simulink model "Simulink_Model"  (R2023b)
settings: Solver=FixedStepAuto  StartTime=0.0  StopTime=100  FixedStep=1e-2  RelTol=1e-3
values from neighbouring files (symbols this model uses):
  A = pi*(diameter/2)^2    (= 0.0706858347058)    [param.m]
  C_d = 0.75    [param.m]
  dm_dt = 3    [param.m]
  h_0 = 0    [param.m]
  m_0 = 200    [param.m]
  m_fuel = 120    [param.m]
  v_exh = 900    [param.m]
undefined symbols (not defined in the file or in its folder): magnitude
libraries: cstblocks x1, simulink x1
settings Model: Creator=Aras Güngöre
settings SolverCC: AlgebraicLoopSolver=TrustRegion
settings DebuggingCC: UnconnectedInputMsg=warning  UnconnectedOutputMsg=warning  UnconnectedLineMsg=warning
settings ModelReferenceCC: EnableRefExpFcnMdlSchedulingChecks=on
settings RTWCC: DLArmComputeVersion=19.05

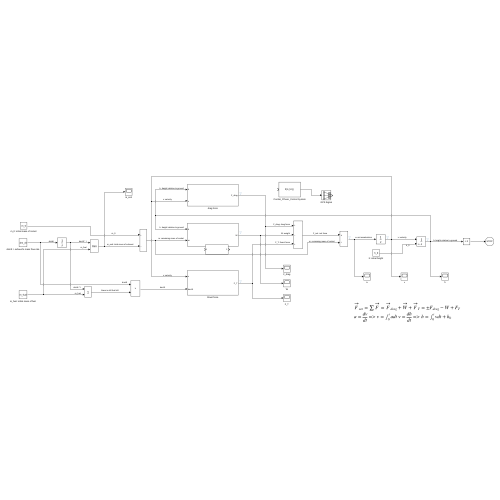
[thumbnail: Simulink's stored preview of the top-level diagram]
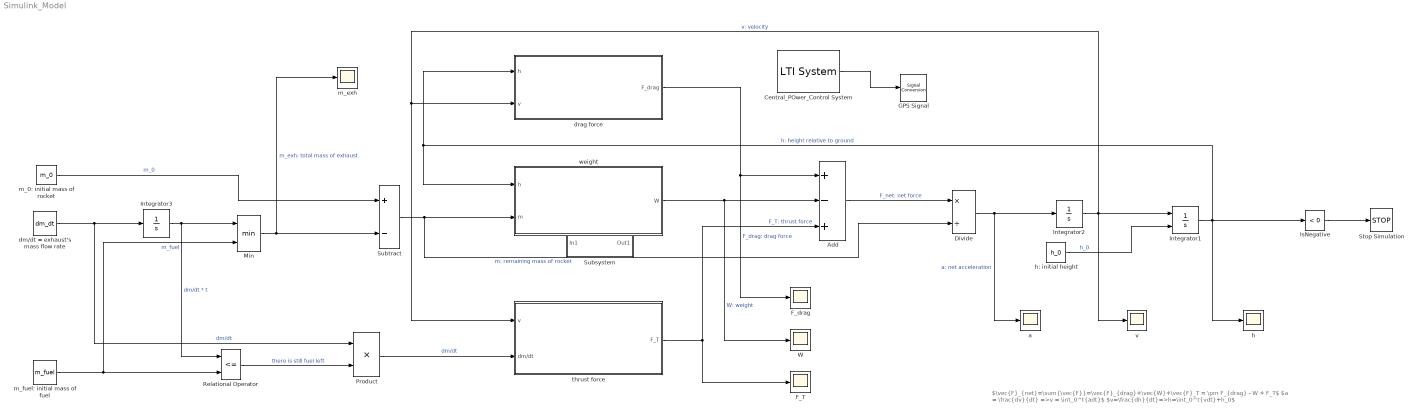
== system Simulink_Model ==
  note: $\vec{F}_{net}=\sum{\vec{F}}=\vec{F}_{drag}+\vec{W}+\vec{F}_T = \pm F_{drag} - W + F_T$
      | $a = \frac{dv}{dt} =>v = \int_0^t{adt}$ $v=\frac{dh}{dt}=>h=\int_0^t{vdt}+h_0$
  Add : Sum  Inputs=+-+
  Central_POwer_Control System : cstblocks/LTI System  sys=tf(1,[1 1])  IC=[]  PadeOrder=0
  Divide : Product  Inputs=*/
  F_T : Scope
  F_drag : Scope
  GPS Signal : SignalConversion  OverrideOpt=off
  Integrator1 : Integrator  InitialConditionSource=external
  Integrator2 : Integrator
  Integrator3 : Integrator
  IsNegative : simulink/Logic and Bit Operations/Compare To Zero  relop=<  OutDataTypeStr=boolean
  Min : MinMax  Inputs=2
  Product : Product
  Relational Operator : RelationalOperator  Operator=<=  OutDataTypeStr=boolean  RndMeth=Simplest  InputSameDT=off
  Stop Simulation : Stop
  Subsystem : Subsystem
  Subtract : Sum  Inputs=+-
  W : Scope
  a : Scope
  dm/dt = exhaust's mass flow rate : Constant  Value=dm_dt
  drag force : Subsystem
  h : Scope
  h: initial height : Constant  Value=h_0
  m_0: initial mass of rocket : Constant  Value=m_0
  m_exh : Scope
  m_fuel: initial mass of fuel : Constant  Value=m_fuel
  thrust force : Subsystem
  v : Scope
  weight : Subsystem
  wires:
  Integrator2/1 -> Integrator1/1, thrust force/1(v), drag force/2(v), v/1  "v: velocity"
  drag force/1(F_drag) -> F_drag/1, Add/1  "F_drag: drag force"
  weight/1(W) -> Add/2, W/1  "W: weight"
  thrust force/1(F_T) -> Add/3, F_T/1  "F_T: thrust force"
  Add/1 -> Divide/1  "F_net: net force"
  Divide/1 -> a/1, Integrator2/1  "a: net acceleration"
  Integrator1/1 -> IsNegative/1, drag force/1(h), weight/1(h), h/1  "h: height relative to ground"
  h: initial height/1 -> Integrator1/2  "h_0"
  IsNegative/1 -> Stop Simulation/1
  m_0: initial mass of rocket/1 -> Subtract/1  "m_0"
  Subtract/1 -> weight/2(m), Divide/2  "m: remaining mass of rocket"
  dm/dt = exhaust's mass flow rate/1 -> Integrator3/1, Product/1  "dm/dt"
  Integrator3/1 -> Min/1, Relational Operator/1  "dm/dt * t"
  m_fuel: initial mass of fuel/1 -> Min/2, Relational Operator/2  "m_fuel"
  Min/1 -> Subtract/2, m_exh/1  "m_exh: total mass of exhaust"
  Relational Operator/1 -> Product/2  "there is still fuel left"
  Product/1 -> thrust force/2(dm/dt)  "dm/dt"
  Central_POwer_Control System/1 -> GPS Signal/1

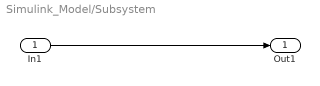
== system Simulink_Model/Subsystem ==
  In1 : Inport
  Out1 : Outport
  wires:
  In1/1 -> Out1/1

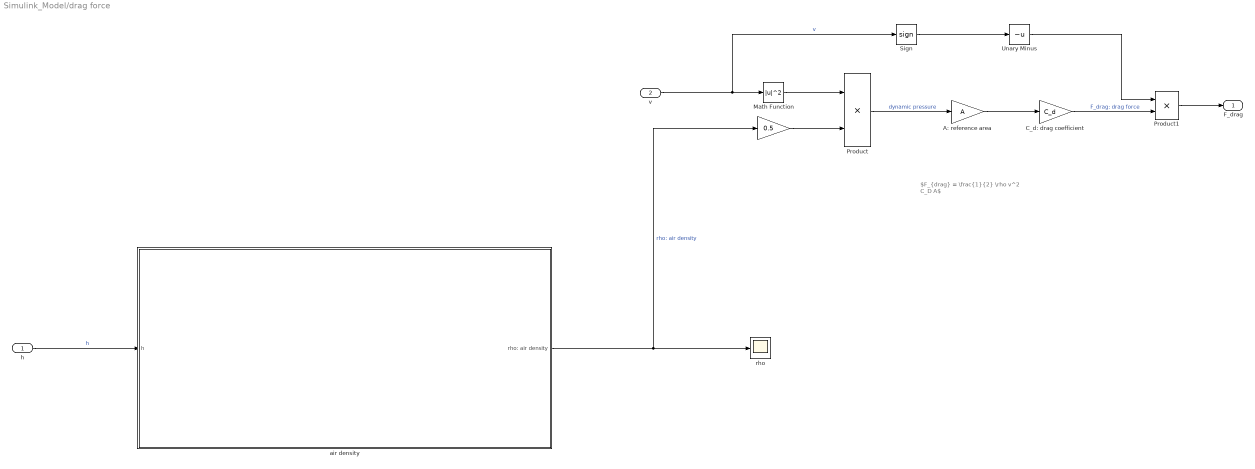
== system Simulink_Model/drag force ==
  note: $F_{drag} = \frac{1}{2} \rho v^2 C_D A$
  h : Inport
  v : Inport  Port=2
  " " : Gain  Gain=0.5
  A: reference area : Gain  Gain=A
  C_d: drag coefficient : Gain  Gain=C_d
  Math Function : Math  Operator=magnitude^2
  Product : Product
  Product1 : Product
  Sign : Signum
  Unary Minus : UnaryMinus
  air density : Subsystem
  rho : Scope
  F_drag : Outport
  wires:
  " "/1 -> Product/2
  v/1 -> Math Function/1, Sign/1  "v"
  Product/1 -> A: reference area/1  "dynamic pressure"
  C_d: drag coefficient/1 -> Product1/2  "F_drag: drag force"
  A: reference area/1 -> C_d: drag coefficient/1
  Math Function/1 -> Product/1
  Sign/1 -> Unary Minus/1
  Product1/1 -> F_drag/1
  Unary Minus/1 -> Product1/1
  h/1 -> air density/1(h)  "h"
  air density/1(rho: air density) -> rho/1, " "/1  "rho: air density"

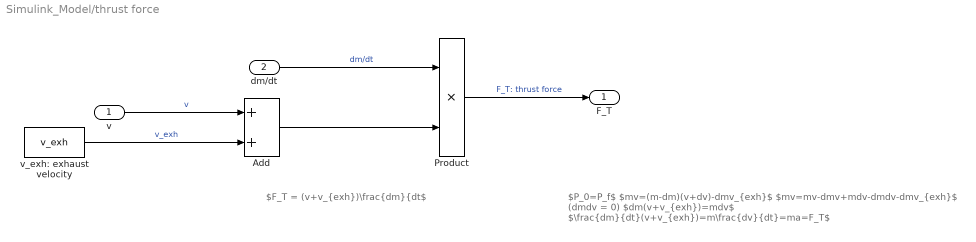
== system Simulink_Model/thrust force ==
  note: $P_0=P_f$
      | $mv=(m-dm)(v+dv)-dmv_{exh}$
      | $mv=mv-dmv+mdv-dmdv-dmv_{exh}$ (dmdv = 0)
      | $dm(v+v_{exh})=mdv$
      | $\frac{dm}{dt}(v+v_{exh})=m\frac{dv}{dt}=ma=F_T$
  note: $F_T = (v+v_{exh})\frac{dm}{dt$
  v : Inport
  dm/dt : Inport  Port=2
  Add : Sum
  Product : Product
  v_exh: exhaust velocity : Constant  Value=v_exh
  F_T : Outport
  wires:
  Product/1 -> F_T/1  "F_T: thrust force"
  dm/dt/1 -> Product/1  "dm/dt"
  v_exh: exhaust velocity/1 -> Add/2  "v_exh"
  v/1 -> Add/1  "v"
  Add/1 -> Product/2

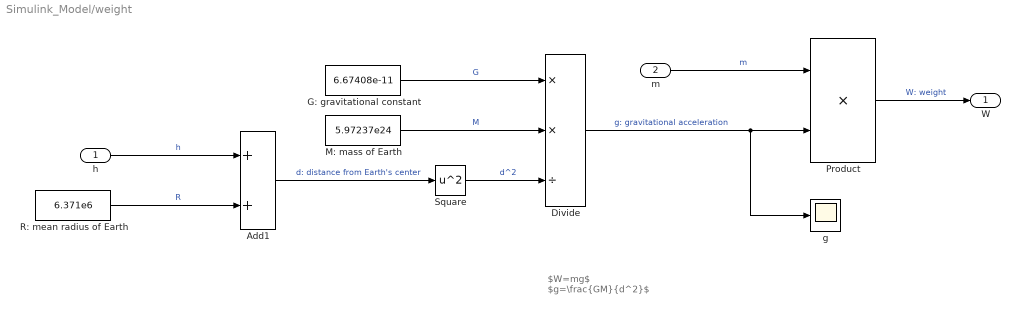
== system Simulink_Model/weight ==
  note: $W=mg$
      | $g=\frac{GM}{d^2}$
  h : Inport
  m : Inport  Port=2
  Add1 : Sum
  Divide : Product  Inputs=**/
  G: gravitational constant : Constant  Value=6.67408e-11
  M: mass of Earth : Constant  Value=5.97237e24
  Product : Product
  R: mean radius of Earth : Constant  Value=6.371e6
  Square : Math  Operator=square
  g : Scope
  W : Outport
  wires:
  m/1 -> Product/1  "m"
  Divide/1 -> g/1, Product/2  "g: gravitational acceleration"
  Product/1 -> W/1  "W: weight"
  G: gravitational constant/1 -> Divide/1  "G"
  M: mass of Earth/1 -> Divide/2  "M"
  Square/1 -> Divide/3  "d^2"
  Add1/1 -> Square/1  "d: distance from Earth's center"
  R: mean radius of Earth/1 -> Add1/2  "R"
  h/1 -> Add1/1  "h"

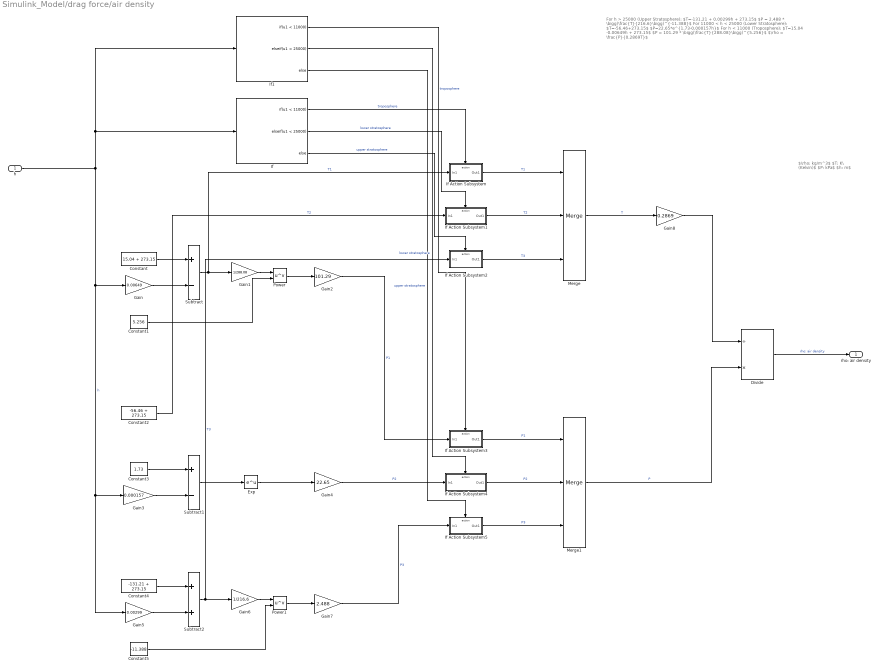
== system Simulink_Model/drag force/air density ==
  note: $\rho: kg/m^3$
      | $T: K\ (Kelvin)$
      | $P: kPa$
      | $h: m$
  note: For h > 25000 (Upper Stratosphere):
      |
      | $T=-131.21 + 0.00299h + 273.15$
      | $P = 2.488 * \bigg(\frac{T}{216.6}\bigg)^{-11.388}$
      |
      | For 11000 < h < 25000 (Lower Stratosphere):
      |
      | $T=-56.46+273.15$
      | $P=22.65*e^{1.73-0.000157h}$
      |
      | For h < 11000 (Troposphere):
      |
      | $T=15.04 -0.00649h + 273.15$
      | $P = 101.29 * \bigg(\frac{T}{288.08}\bigg)^{5.256}$
      |
      | $\rho = \frac{P}{0.2869T}$
  h : Inport
  Constant : Constant  Value=15.04 + 273.15
  Constant1 : Constant  Value=5.256
  Constant2 : Constant  Value=-56.46 + 273.15
  Constant3 : Constant  Value=1.73
  Constant4 : Constant  Value=-131.21 + 273.15
  Constant5 : Constant  Value=-11.388
  Divide : Product  Inputs=/*
  Exp : Math
  Gain : Gain  Gain=0.00649
  Gain1 : Gain  Gain=1/288.08
  Gain2 : Gain  Gain=101.29
  Gain3 : Gain  Gain=0.000157
  Gain4 : Gain  Gain=22.65
  Gain5 : Gain  Gain=0.00299
  Gain6 : Gain  Gain=1/216.6
  Gain7 : Gain  Gain=2.488
  Gain8 : Gain  Gain=0.2869
  If : If  IfExpression=u1 < 11000  ElseIfExpressions=u1 < 25000
  If Action Subsystem : Subsystem  TreatAsAtomicUnit=on
  If Action Subsystem1 : Subsystem  TreatAsAtomicUnit=on
  If Action Subsystem2 : Subsystem  TreatAsAtomicUnit=on
  If Action Subsystem3 : Subsystem  TreatAsAtomicUnit=on
  If Action Subsystem4 : Subsystem  TreatAsAtomicUnit=on
  If Action Subsystem5 : Subsystem  TreatAsAtomicUnit=on
  If1 : If  IfExpression=u1 < 11000  ElseIfExpressions=u1 < 25000
  Merge : Merge  Inputs=3
  Merge1 : Merge  Inputs=3
  Power : Math  Operator=pow
  Power1 : Math  Operator=pow
  Subtract : Sum  Inputs=+-
  Subtract1 : Sum  Inputs=+-
  Subtract2 : Sum
  rho: air density : Outport
  wires:
  Gain2/1 -> If Action Subsystem3/1(In1)  "P1"
  Subtract/1 -> Gain1/1, If Action Subsystem/1(In1)  "T1"
  If Action Subsystem4/1(Out1) -> Merge1/2  "P2"
  If Action Subsystem5/1(Out1) -> Merge1/3  "P3"
  If/3 -> If Action Subsystem2/Action  "upper stratosphere"
  If Action Subsystem/1(Out1) -> Merge/1  "T1"
  Constant2/1 -> If Action Subsystem1/1(In1)  "T2"
  Gain3/1 -> Subtract1/2
  Merge1/1 -> Divide/2  "P"
  h/1 -> Gain/1, Gain3/1, Gain5/1, If/1, If1/1  "h"
  Merge/1 -> Gain8/1  "T"
  Gain1/1 -> Power/1
  Constant3/1 -> Subtract1/1
  Exp/1 -> Gain4/1
  Constant4/1 -> Subtract2/1
  Subtract1/1 -> Exp/1
  If/2 -> If Action Subsystem1/Action  "lower stratosphere"
  If Action Subsystem2/1(Out1) -> Merge/3  "T3"
  Subtract2/1 -> Gain6/1, If Action Subsystem2/1(In1)  "T3"
  Gain4/1 -> If Action Subsystem4/1(In1)  "P2"
  Constant1/1 -> Power/2
  Gain/1 -> Subtract/2
  Gain5/1 -> Subtract2/2
  Power/1 -> Gain2/1
  Gain6/1 -> Power1/1
  Power1/1 -> Gain7/1
  Constant5/1 -> Power1/2
  Constant/1 -> Subtract/1
  If/1 -> If Action Subsystem/Action  "troposphere"
  If Action Subsystem3/1(Out1) -> Merge1/1  "P1"
  Gain8/1 -> Divide/1
  Gain7/1 -> If Action Subsystem5/1(In1)  "P3"
  Divide/1 -> rho: air density/1  "rho: air density"
  If Action Subsystem1/1(Out1) -> Merge/2  "T2"
  If1/2 -> If Action Subsystem4/Action  "lower stratosphere"
  If1/3 -> If Action Subsystem5/Action  "upper stratosphere"
  If1/1 -> If Action Subsystem3/Action  "troposphere"

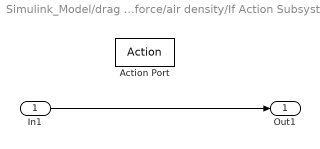
== system Simulink_Model/drag force/air density/If Action Subsystem ==
  In1 : Inport
  Action Port : ActionPort  ActionPortLabel=if(u1 < 11000)
  Out1 : Outport
  wires:
  In1/1 -> Out1/1

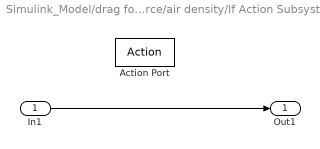
== system Simulink_Model/drag force/air density/If Action Subsystem1 ==
  In1 : Inport
  Action Port : ActionPort  ActionPortLabel=elseif(u1 < 25000)
  Out1 : Outport
  wires:
  In1/1 -> Out1/1

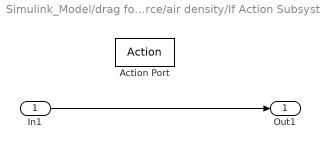
== system Simulink_Model/drag force/air density/If Action Subsystem2 ==
  In1 : Inport
  Action Port : ActionPort  ActionPortLabel=else
  Out1 : Outport
  wires:
  In1/1 -> Out1/1

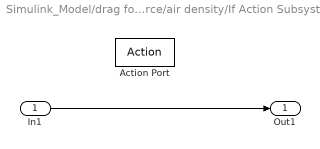
== system Simulink_Model/drag force/air density/If Action Subsystem3 ==
  In1 : Inport
  Action Port : ActionPort  ActionPortLabel=if(u1 < 11000)
  Out1 : Outport
  wires:
  In1/1 -> Out1/1

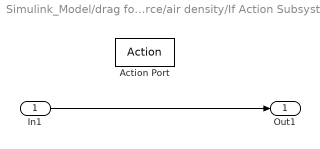
== system Simulink_Model/drag force/air density/If Action Subsystem4 ==
  In1 : Inport
  Action Port : ActionPort  ActionPortLabel=elseif(u1 < 25000)
  Out1 : Outport
  wires:
  In1/1 -> Out1/1

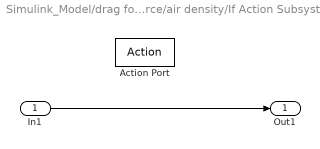
== system Simulink_Model/drag force/air density/If Action Subsystem5 ==
  In1 : Inport
  Action Port : ActionPort  ActionPortLabel=else
  Out1 : Outport
  wires:
  In1/1 -> Out1/1
